simulink model "Pacejka_Lateral_Tyre_Model"  (R2025a)
settings: Solver=FixedStepAuto  StartTime=0.0  StopTime=10.0  FixedStep=0.01  RelTol=1e-3
values from neighbouring files (symbols this model uses):
  a1 = -1e-5    (= -1e-05)    [Pacejka_Lateral_Parameters.m]
  a2 = 1.25    [Pacejka_Lateral_Parameters.m]
  B = 0.1453    [Pacejka_Lateral_Parameters.m]
  C = 1.5511    [Pacejka_Lateral_Parameters.m]
settings Model: Creator=g.m.morjaria  LastModifiedBy=g.m.morjaria

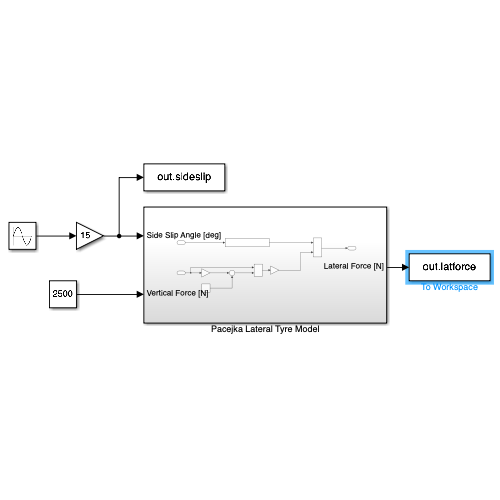
[thumbnail: Simulink's stored preview of the top-level diagram]
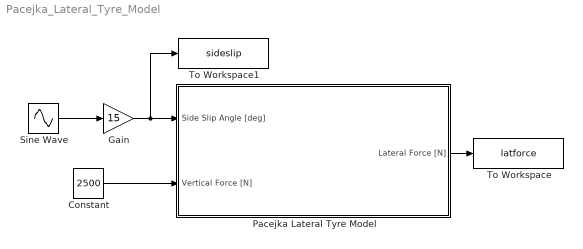
== system Pacejka_Lateral_Tyre_Model ==
  Constant : Constant  Value=2500
  Gain : Gain  Gain=15
  Pacejka Lateral Tyre Model : Subsystem
  Sine Wave : Sin  SampleTime=0
  To Workspace : ToWorkspace  VariableName=latforce  SaveFormat=Timeseries  SampleTime=-1
  To Workspace1 : ToWorkspace  VariableName=sideslip  SaveFormat=Timeseries  SampleTime=-1
  wires:
  Constant/1 -> Pacejka Lateral Tyre Model/2(Vertical Force [N])
  Sine Wave/1 -> Gain/1
  Gain/1 -> To Workspace1/1, Pacejka Lateral Tyre Model/1(Side Slip Angle [deg])
  Pacejka Lateral Tyre Model/1(Lateral Force [N]) -> To Workspace/1

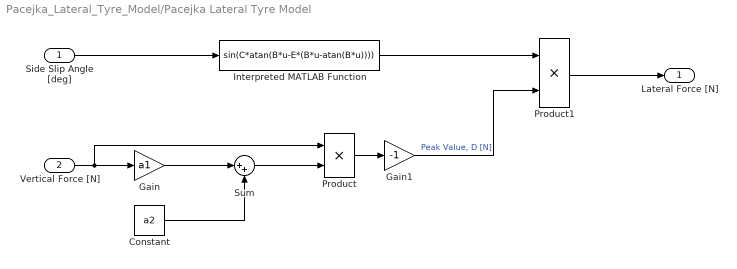
== system Pacejka_Lateral_Tyre_Model/Pacejka Lateral Tyre Model ==
  Side Slip Angle [deg] : Inport
  Vertical Force [N] : Inport  Port=2
  Constant : Constant  Value=a2
  Gain : Gain  Gain=a1
  Gain1 : Gain  Gain=-1
  Interpreted MATLAB Function : MATLABFcn  MATLABFcn=sin(C*atan(B*u-E*(B*u-atan(B*u))))
  Product : Product
  Product1 : Product
  Sum : Sum  Inputs=|++
  Lateral Force [N] : Outport
  wires:
  Vertical Force [N]/1 -> Product/1, Gain/1
  Gain/1 -> Sum/1
  Constant/1 -> Sum/2
  Sum/1 -> Product/2
  Product/1 -> Gain1/1
  Gain1/1 -> Product1/2  "Peak Value, D [N]"
  Side Slip Angle [deg]/1 -> Interpreted MATLAB Function/1
  Interpreted MATLAB Function/1 -> Product1/1
  Product1/1 -> Lateral Force [N]/1
